simulink model "mech_car_kinematics"  (Simulink 7.1)
settings: Solver=ode45  StartTime=0.0  StopTime=10  RelTol=1e-3
PreLoadFcn:
  | % Initialize structures
  | chassis = struct() ;
  | wheelhub = struct() ;
  | suspension = struct() ;
  | wheel = struct() ;
  | 
  | % Defualt chassis/double wishbone mounting points
  | chassis.mass = 600 ;
  | chassis.upperfront = [0 0 0] ;
  | chassis.upperback = [-0.4 0 0] ;
  | chassis.lowerfront = [0 0 -0.5] ;
  | chassis.lowerback = [-0.4 0 -0.45] ;
  | chassis.steering = [0.12 0 -0.3] ;
  | chassis.suspension = [0 0 0.3] ;
  | 
  | % Default wheel hub/double wishbone mounting points
  | wheelhub.upper = [-0.2 0.55 0] ;
  | wheelhub.lower = [-0.2 0.55 -0.5] ;
  | wheelhub.steering = [0.05 0.5 -0.3] ;
  | wheelhub.suspension = [-0.2 0.55 -0.5] ;
  | 
  | % Default suspension parameters
  | suspension.ks = 16000 ;
  | suspension.bs = 1100 ;
  | suspension.Ls = 1.2 ;
  | 
  | % Defualt wheel parameters
  | wheel.radius = 0.3;
  | wheel.mass = 45 ;
  | wheel.inertia = [0.52 0 0;0 1 0;0 0 0.52]*2.5;
InitFcn:
  | set_param([gcs '/WORLD/Machine Environment'], 'AnalysisType', 'Kinematics');
StopFcn:
  | % Script to plot the bump steer properties of a suspension system
  | 
  | appDataName = 'mech_car_Kin_Steering_data';
  | figInfo.pos = [20   288   409   413];
  | figInfo.title = 'Steering angle versus CG height';
  | figInfo.xlabel = 'CG Height (m)';
  | figInfo.ylabel = 'Steering Angle (deg)';
  | mech_car_handling_fig_mgr('init',appDataName,figInfo);
  | modelFigure = getappdata(0,appDataName);
  | plot(-WHEEL.signals.values(:,1),STEER.signals.values,'Parent',modelFigure.axesH);
  | 
  | appDataName = 'mech_car_Kin_CamberAng_data';
  | figInfo.pos = [436   288   451   413];
  | figInfo.title = 'Camber angle versus CG height';
  | figInfo.xlabel = 'CG Height (m)';
  | figInfo.ylabel = 'Camber Angle (deg)';
  | mech_car_handling_fig_mgr('init',appDataName,figInfo);
  | modelFigure = getappdata(0,appDataName);
  | plot(-WHEEL.signals.values(:,1),CAMBER.signals.values,'Parent',modelFigure.axesH);
  | 
  | appDataName = 'mech_car_Kin_CasterAng_data';
  | figInfo.pos = [20   -154   411   369];
  | figInfo.title = 'Caster angle versus CG height';
  | figInfo.xlabel = 'CG Height (m)';
  | figInfo.ylabel = 'Caster Angle (deg)';
  | mech_car_handling_fig_mgr('init',appDataName,figInfo);
  | modelFigure = getappdata(0,appDataName);
  | plot(-WHEEL.signals.values(:,1),CASTER.signals.values,'Parent',modelFigure.axesH);
libraries: mblibv1 x27, mech_car_library x8, simulink x4
Description:
  | Car Suspension Kinematics
  | 
  | When designing a suspension system, it is important to know the effect of travel on the wheel alignment. This is measured by Camber, Steering, and Caster angles.
  | 
  | This quarter car model uses the SimMechanics Kinematics mode to measure these angles for a range of CG heights.
  | 
  | The Car parameters are defined in the PreLoad function of the model.
CloseFcn:
  | mech_car_handling_fig_mgr('destroy','mech_car_Kin_Steering_data');
  | mech_car_handling_fig_mgr('destroy','mech_car_Kin_CamberAng_data');
  | mech_car_handling_fig_mgr('destroy','mech_car_Kin_CasterAng_data');
settings Model: Creator=arnav  LastModifiedBy=batserve  BufferReuse=off
settings OptimizationCC: InlineParams=on  BufferReuse=off
settings DebuggingCC: SaveWithParameterizedLinksMsg=none  SignalResolutionControl=TryResolveAllWithWarning  SolverPrmCheckMsg=none  MultiTaskDSMMsg=warning  MultiTaskCondExecSysMsg=none  StrictBusMsg=None
settings HardwareCC: TargetBitPerLong=64  TargetEndianess=LittleEndian  TargetWordSize=64  TargetHWDeviceType=MATLAB Host  ProdEqTarget=off
settings RTWCC: SystemTargetFile=rsim.tlc  TemplateMakefile=rsim_default_tmf  Description=Rapid Simulation Target  ProcessScript=rsim_make_rtw_hook  IncludeERTFirstTime=on
settings RSimTargetCC: TargetFcnLib=ansi_tfl_tmw.mat  TargetFunctionLibrary=ANSI_C  IsPILTarget=off  EnableShiftOperators=on  PortableWordSizes=off
settings SimMechanicsCC: WarnOnRedundantConstraints=off  VisOnUpdateDiagram=on

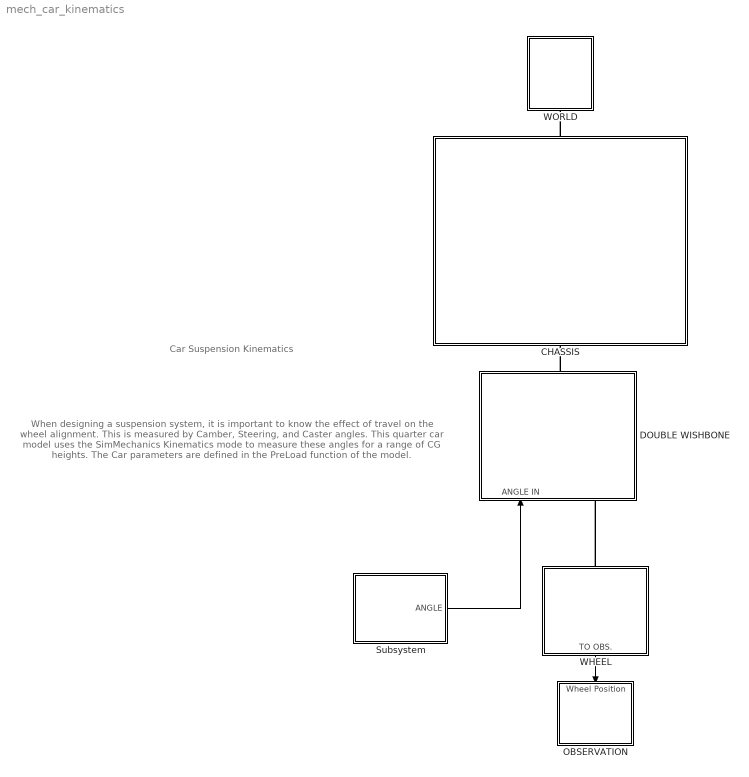
== system mech_car_kinematics ==
  note: When designing a suspension system, it is important
      | to know the effect of travel on the wheel alignment.
      | This is measured by Camber, Steering, and Caster angles.
      |
      | This quarter car model uses the SimMechanics Kinematics mode
      | to measure these angles for a range of CG heights.
      |
      | The Car parameters are defined in the PreLoad function of the model.
  note: Car Suspension Kinematics
  CHASSIS : Subsystem  Orientation=down  mask{chassis_mass=chassis.mass}
      mask prompts: chassis_mass "Quarter Car Chassis Mass"
      mask Display: image(imread('chassis.jpg'))
  DOUBLE WISHBONE : Subsystem  Orientation=up  mask{Chas_Up_Front=chassis.upperfront, Chas_Up_Back=chassis.upperback, Chas_Low_Front=chassis.lowerfront, Chas_Low_Back=chassis.lowerback, Chas_Steer=chassis.steering, Chas_Susp=chassis.suspension, Hub_Up=wheelhub.upper, Hub_Low=wheelhub.lower, Hub_Steer=wheelhub.steering, Hub_Susp=wheelhub.suspension, suspension_ks=suspension.ks, suspension_Ls=suspension.Ls, suspension_bs=suspension.bs}
      mask prompts: Chas_Up_Front "Chassis Upper Front Mounting"; Chas_Up_Back "Chassis Upper Back"; Chas_Low_Front "Chassis Lower Front"; Chas_Low_Back "Chassis Lower Back"; Chas_Steer "Chassis Steering Arm"; Chas_Susp "Chassis Suspension"; Hub_Up "Hub Upper"; Hub_Low "Hub Lower"; Hub_Steer "Hub Steering Arm"; Hub_Susp "Hub Suspension"; suspension_ks "Suspension Spring Stiffness"; suspension_Ls "Suspension Spring Natural Length"; suspension_bs "Suspension Damping Constant"
      mask Display: image(imread('double_wishbone.jpg'))
  OBSERVATION : Subsystem  Orientation=down
      mask Display: image(imread('view.jpg'))
  Subsystem : Subsystem
      mask Display: image(imread('spanner.jpg'))
  WHEEL : Subsystem  Orientation=down  mask{wheel_mass=wheel.mass, wheel_radius=wheel.radius, wheel_inertia=wheel.inertia}
      mask prompts: wheel_mass "Wheel Mass"; wheel_radius "Wheel Radius"; wheel_inertia "Wheel Inertia"
      mask Display: image(imread('wheel.jpg'))
  WORLD : Subsystem  Orientation=down
      mask Display: image(imread('sky.jpg'))
  wires:
  Subsystem/1(ANGLE) -> DOUBLE WISHBONE/1(ANGLE IN)
  WHEEL/1(TO OBS.) -> OBSERVATION/1(Wheel Position)
  connections:
  CHASSIS/LConn1 -- WORLD/RConn1
  WHEEL/LConn1 -- DOUBLE WISHBONE/LConn1
  DOUBLE WISHBONE/RConn1 -- CHASSIS/RConn1

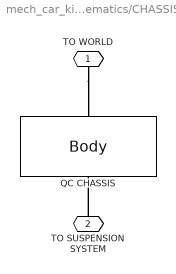
== system mech_car_kinematics/CHASSIS ==
  QC CHASSIS : mblibv1/Bodies/Body  Orientation=down  DialogController=MECH.DynMechDlgSource  PhysicalDomain=mechanical  SubClassName=Unknown  LeftPortType=workingframe  RightPortType=workingframe  LConnTagsString=CS1  RConnTagsString=CS2  DialogClass=MechanicalBodyBlock  Mass=chassis_mass  MassUnits=kg  InertiaUnits=kg*m^2  Inertia=diag([1 1 0.008])*10  Shape=Cylinder  ShapeDims=[1 1]  ShapeUnits=m  ShapeUse=false  Density=1  DensityUnits=kg/m^3  DensityUse=false  GraphicsMode=1  BodyColor=[0.5 0.5 0.5]  GraphicsObj=[]  AttachedToCS=1  CG=Left$CG$[0 0 -0.5]$CS1$CS1$m$[0 0 0]$EULER X-Y-Z$deg$WORLD$false  WorkingFrames=Left$CS1$[0 0 0]$ADJOINING$ADJOINING$m$[0 0 0]$EULER X-Y-Z$deg$WORLD$true#Right$CS2$[0 0 -1]$CS1$CS1$m$[0 0 0]$EULER X-Y-Z$deg$WORLD$true  CGPos=[0 0 -0.5]  CGRot=[0 0 0]  CS0Pos=[]  CS0Rot=[]  CS1Pos=[0 0 0]  CS1Rot=[0 0 0]  CS2Pos=[0 0 -1]  CS2Rot=[0 0 0]  CS3Pos=[]  CS3Rot=[]  CS4Pos=[]  CS4Rot=[]  CS5Pos=[]  CS5Rot=[]  CS6Pos=[]  CS6Rot=[]  CS7Pos=[]  CS7Rot=[]  CS8Pos=[]  CS8Rot=[]  CS9Pos=[]  CS9Rot=[]  CS10Pos=[]  CS10Rot=[]  CS11Pos=[]  CS11Rot=[]  CS12Pos=[]  CS12Rot=[]  CS13Pos=[]  CS13Rot=[]  CS14Pos=[]  CS14Rot=[]  CS15Pos=[]  CS15Rot=[]  CS16Pos=[]  CS16Rot=[]  CS17Pos=[]  CS17Rot=[]  CS18Pos=[]  CS18Rot=[]  CS19Pos=[]  CS19Rot=[]  CS20Pos=[]  CS20Rot=[]
  TO WORLD : PMIOPort  Orientation=down  Port=1  Side=Left
  TO SUSPENSION SYSTEM : PMIOPort  Orientation=up  Port=2  Side=Right
  connections:
  TO WORLD/RConn1 -- QC CHASSIS/LConn1
  TO SUSPENSION SYSTEM/RConn1 -- QC CHASSIS/RConn1

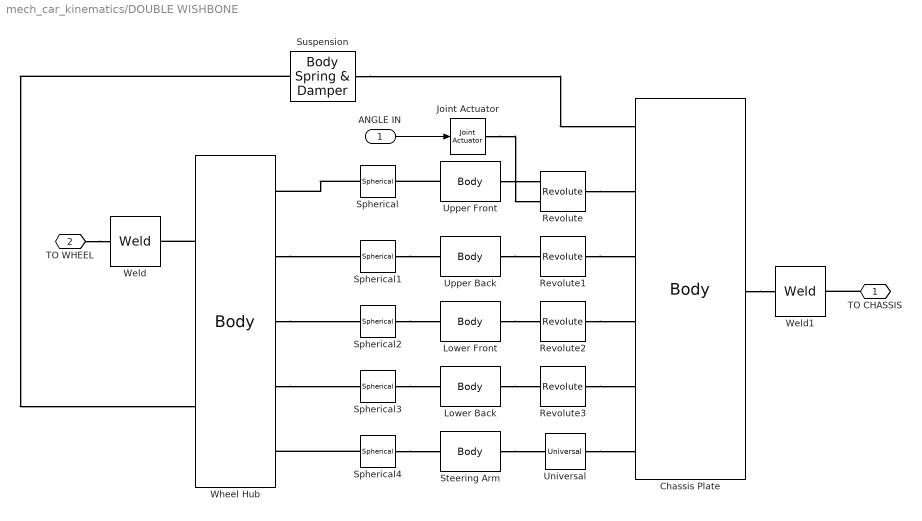
== system mech_car_kinematics/DOUBLE WISHBONE ==
  ANGLE IN : Inport  OutDataType=sfix(16)  OutScaling=2^0
  Chassis Plate : mblibv1/Bodies/Body  DialogController=MECH.DynMechDlgSource  PhysicalDomain=mechanical  SubClassName=Unknown  LeftPortType=workingframe  RightPortType=workingframe  LConnTagsString=CS1|CS3|CS2|CS5|CS6|CS7  RConnTagsString=CS4  DialogClass=MechanicalBodyBlock  Mass=0.1  MassUnits=kg  InertiaUnits=kg*m^2  Inertia=[0.5005 0 0;0 1 0;0 0 0.5005]/100  Shape=Cylinder  ShapeDims=[1 1]  ShapeUnits=m  ShapeUse=false  Density=1  DensityUnits=kg/m^3  DensityUse=false  GraphicsMode=1  BodyColor=[0.5 0.5 0.5]  GraphicsObj=[]  AttachedToCS=1  CG=Right$CG$[0 0 0]$CS4$CS4$m$[0 0 0]$EULER X-Y-Z$deg$WORLD$false  WorkingFrames=Right$CS4$[0 0 0]$ADJOINING$ADJOINING$m$[0 0 0]$EULER X-Y-Z$deg$WORLD$true#Left$CS1$Chas_Susp$CS4$CS4$m$[0 0 0]$EULER X-Y-Z$deg$WORLD$true#Left$CS3$Chas_Up_Front$CS4$CS4$m$[0 0 0]$EULER X-Y-Z$deg$WORLD$true#Left$CS2$Chas_Up_Back$CS4$CS4$m$[0 0 0]$EULER X-Y-Z$deg$WORLD$true#Left$CS5$Chas_Low_Front$CS4$CS4$m$[0 0 0]$EULER X-Y-Z$deg$WORLD$true#Left$CS6$Chas_Low_Back$CS4$CS4$m$[0 0 0]$EULER X-Y-Z$deg$WORLD$true#Left$CS7$Chas_Steer$CS4$CS4$m$[0 0 0]$EULER X-Y-Z$deg$WORLD$true  CGPos=[0 0 0]  CGRot=[0 0 0]  CS0Pos=[]  CS0Rot=[]  CS1Pos=Chas_Susp  CS1Rot=[0 0 0]  CS2Pos=Chas_Up_Back  CS2Rot=[0 0 0]  CS3Pos=Chas_Up_Front  CS3Rot=[0 0 0]  CS4Pos=[0 0 0]  CS4Rot=[0 0 0]  CS5Pos=Chas_Low_Front  CS5Rot=[0 0 0]  CS6Pos=Chas_Low_Back  CS6Rot=[0 0 0]  CS7Pos=Chas_Steer  CS7Rot=[0 0 0]  CS8Pos=[]  CS8Rot=[]  CS9Pos=[]  CS9Rot=[]  CS10Pos=[]  CS10Rot=[]  CS11Pos=[]  CS11Rot=[]  CS12Pos=[]  CS12Rot=[]  CS13Pos=[]  CS13Rot=[]  CS14Pos=[]  CS14Rot=[]  CS15Pos=[]  CS15Rot=[]  CS16Pos=[]  CS16Rot=[]  CS17Pos=[]  CS17Rot=[]  CS18Pos=[]  CS18Rot=[]  CS19Pos=[]  CS19Rot=[]  CS20Pos=[]  CS20Rot=[]
  Joint Actuator : mblibv1/Sensors &  Actuators/Joint Actuator  DialogController=MECH.DynMechDlgSource  SystemSampleTime=-1  PhysicalDomain=Mechanical  PortType=blob  ActuationStyle=Motion  AngleUnits=rad  ArcVelocityUnits=rad/s  ArcAccelerationUnits=rad/s^2  CoordPositionUnits=m  VelocityUnits=m/s  AccelerationUnits=m/s^2  ForceUnits=N  TorqueUnits=N-m  ActiveIO=on  Width=3  DialogClass=MechanicalActuatorBlock  Primitive=R1  ReferenceFrame=Absolute (INERTIAL)
  Lower Back : mblibv1/Bodies/Body  DialogController=MECH.DynMechDlgSource  PhysicalDomain=mechanical  SubClassName=Unknown  LeftPortType=workingframe  RightPortType=workingframe  LConnTagsString=CS1  RConnTagsString=CS2  DialogClass=MechanicalBodyBlock  Mass=7  MassUnits=kg  InertiaUnits=kg*m^2  Inertia=diag([0.008 1 1])/7.8  Shape=Cylinder  ShapeDims=[1 1]  ShapeUnits=m  ShapeUse=false  Density=1  DensityUnits=kg/m^3  DensityUse=false  GraphicsMode=1  BodyColor=[0.5 0.5 0.5]  GraphicsObj=[]  AttachedToCS=1  CG=Left$CG$0.5*(Hub_Low - Chas_Low_Back)$CS2$CS2$m$[0 0 -110]$EULER X-Y-Z$deg$WORLD$false  WorkingFrames=Left$CS1$Hub_Low - Chas_Low_Back$CS2$CS2$m$[0 0 0]$EULER X-Y-Z$deg$WORLD$true#Right$CS2$[0 0 0]$ADJOINING$ADJOINING$m$[0 0 0]$EULER X-Y-Z$deg$WORLD$true  CGPos=0.5*(Hub_Low - Chas_Low_Back)  CGRot=[0 0 -110]  CS0Pos=[]  CS0Rot=[]  CS1Pos=Hub_Low - Chas_Low_Back  CS1Rot=[0 0 0]  CS2Pos=[0 0 0]  CS2Rot=[0 0 0]  CS3Pos=[]  CS3Rot=[]  CS4Pos=[]  CS4Rot=[]  CS5Pos=[]  CS5Rot=[]  CS6Pos=[]  CS6Rot=[]  CS7Pos=[]  CS7Rot=[]  CS8Pos=[]  CS8Rot=[]  CS9Pos=[]  CS9Rot=[]  CS10Pos=[]  CS10Rot=[]  CS11Pos=[]  CS11Rot=[]  CS12Pos=[]  CS12Rot=[]  CS13Pos=[]  CS13Rot=[]  CS14Pos=[]  CS14Rot=[]  CS15Pos=[]  CS15Rot=[]  CS16Pos=[]  CS16Rot=[]  CS17Pos=[]  CS17Rot=[]  CS18Pos=[]  CS18Rot=[]  CS19Pos=[]  CS19Rot=[]  CS20Pos=[]  CS20Rot=[]
  Lower Front : mblibv1/Bodies/Body  DialogController=MECH.DynMechDlgSource  PhysicalDomain=mechanical  SubClassName=Unknown  LeftPortType=workingframe  RightPortType=workingframe  LConnTagsString=CS1  RConnTagsString=CS2  DialogClass=MechanicalBodyBlock  Mass=7  MassUnits=kg  InertiaUnits=kg*m^2  Inertia=diag([0.008 1 1])/7.8  Shape=Cylinder  ShapeDims=[1 1]  ShapeUnits=m  ShapeUse=false  Density=1  DensityUnits=kg/m^3  DensityUse=false  GraphicsMode=1  BodyColor=[0.5 0.5 0.5]  GraphicsObj=[]  AttachedToCS=1  CG=Left$CG$0.5*(Hub_Low - Chas_Low_Front)$CS2$CS2$m$[0 0 -70]$EULER X-Y-Z$deg$WORLD$false  WorkingFrames=Left$CS1$Hub_Low - Chas_Low_Front$CS2$CS2$m$[0 0 0]$EULER X-Y-Z$deg$WORLD$true#Right$CS2$[0 0 0]$ADJOINING$ADJOINING$m$[0 0 0]$EULER X-Y-Z$deg$WORLD$true  CGPos=0.5*(Hub_Low - Chas_Low_Front)  CGRot=[0 0 -70]  CS0Pos=[]  CS0Rot=[]  CS1Pos=Hub_Low - Chas_Low_Front  CS1Rot=[0 0 0]  CS2Pos=[0 0 0]  CS2Rot=[0 0 0]  CS3Pos=[]  CS3Rot=[]  CS4Pos=[]  CS4Rot=[]  CS5Pos=[]  CS5Rot=[]  CS6Pos=[]  CS6Rot=[]  CS7Pos=[]  CS7Rot=[]  CS8Pos=[]  CS8Rot=[]  CS9Pos=[]  CS9Rot=[]  CS10Pos=[]  CS10Rot=[]  CS11Pos=[]  CS11Rot=[]  CS12Pos=[]  CS12Rot=[]  CS13Pos=[]  CS13Rot=[]  CS14Pos=[]  CS14Rot=[]  CS15Pos=[]  CS15Rot=[]  CS16Pos=[]  CS16Rot=[]  CS17Pos=[]  CS17Rot=[]  CS18Pos=[]  CS18Rot=[]  CS19Pos=[]  CS19Rot=[]  CS20Pos=[]  CS20Rot=[]
  Revolute : mblibv1/Joints/Revolute  DialogController=MECH.DynMechDlgSource  PhysicalDomain=mechanical  SubClassName=Unknown  LeftPortType=blob  RightPortType=blob  LConnTagsString=__newl0|SA1  RConnTagsString=__newr0  NumSAPorts=1  CutJoint=off  MarkAsCut=off  Primitives=revolute  PrimitiveProps=R1$WORLD$Chas_Up_Front - Chas_Up_Back$revolute  DialogClass=JointBlock  R1Axis=Chas_Up_Front - Chas_Up_Back
  Revolute1 : mblibv1/Joints/Revolute  DialogController=MECH.DynMechDlgSource  PhysicalDomain=mechanical  SubClassName=Unknown  LeftPortType=blob  RightPortType=blob  LConnTagsString=__newl0  RConnTagsString=__newr0  NumSAPorts=0  CutJoint=on  MarkAsCut=off  Primitives=revolute  PrimitiveProps=R1$WORLD$Chas_Up_Front - Chas_Up_Back$revolute  DialogClass=JointBlock  R1Axis=Chas_Up_Front - Chas_Up_Back
  Revolute2 : mblibv1/Joints/Revolute  DialogController=MECH.DynMechDlgSource  PhysicalDomain=mechanical  SubClassName=Unknown  LeftPortType=blob  RightPortType=blob  LConnTagsString=__newl0  RConnTagsString=__newr0  NumSAPorts=0  CutJoint=off  MarkAsCut=off  Primitives=revolute  PrimitiveProps=R1$WORLD$Chas_Low_Front-Chas_Low_Back$revolute  DialogClass=JointBlock  R1Axis=Chas_Low_Front-Chas_Low_Back
  Revolute3 : mblibv1/Joints/Revolute  DialogController=MECH.DynMechDlgSource  PhysicalDomain=mechanical  SubClassName=Unknown  LeftPortType=blob  RightPortType=blob  LConnTagsString=__newl0  RConnTagsString=__newr0  NumSAPorts=0  CutJoint=off  MarkAsCut=off  Primitives=revolute  PrimitiveProps=R1$WORLD$Chas_Low_Front - Chas_Low_Back$revolute  DialogClass=JointBlock  R1Axis=Chas_Low_Front - Chas_Low_Back
  Spherical : mblibv1/Joints/Spherical  DialogController=MECH.DynMechDlgSource  PhysicalDomain=mechanical  SubClassName=Unknown  LeftPortType=blob  RightPortType=blob  LConnTagsString=__newl0  RConnTagsString=__newr0  NumSAPorts=0  CutJoint=off  MarkAsCut=off  Primitives=spherical  PrimitiveProps=S$INERTIAL$[0 0 0]$spherical  DialogClass=JointBlock  SAxis=[0 0 0]
  Spherical1 : mblibv1/Joints/Spherical  DialogController=MECH.DynMechDlgSource  PhysicalDomain=mechanical  SubClassName=Unknown  LeftPortType=blob  RightPortType=blob  LConnTagsString=__newl0  RConnTagsString=__newr0  NumSAPorts=0  CutJoint=off  MarkAsCut=off  Primitives=spherical  PrimitiveProps=S$WORLD$[0 0 0]$spherical  DialogClass=JointBlock  SAxis=[0 0 0]
  Spherical2 : mblibv1/Joints/Spherical  DialogController=MECH.DynMechDlgSource  PhysicalDomain=mechanical  SubClassName=Unknown  LeftPortType=blob  RightPortType=blob  LConnTagsString=__newl0  RConnTagsString=__newr0  NumSAPorts=0  CutJoint=off  MarkAsCut=off  Primitives=spherical  PrimitiveProps=S$WORLD$[0 0 0]$spherical  DialogClass=JointBlock  SAxis=[0 0 0]
  Spherical3 : mblibv1/Joints/Spherical  DialogController=MECH.DynMechDlgSource  PhysicalDomain=mechanical  SubClassName=Unknown  LeftPortType=blob  RightPortType=blob  LConnTagsString=__newl0  RConnTagsString=__newr0  NumSAPorts=0  CutJoint=on  MarkAsCut=off  Primitives=spherical  PrimitiveProps=S$WORLD$[0 0 0]$spherical  DialogClass=JointBlock  SAxis=[0 0 0]
  Spherical4 : mblibv1/Joints/Spherical  DialogController=MECH.DynMechDlgSource  PhysicalDomain=mechanical  SubClassName=Unknown  LeftPortType=blob  RightPortType=blob  LConnTagsString=__newl0  RConnTagsString=__newr0  NumSAPorts=0  CutJoint=off  MarkAsCut=off  Primitives=spherical  PrimitiveProps=S$INERTIAL$[0 0 0]$spherical  DialogClass=JointBlock  SAxis=[0 0 0]
  Steering Arm : mblibv1/Bodies/Body  DialogController=MECH.DynMechDlgSource  PhysicalDomain=mechanical  SubClassName=Unknown  LeftPortType=workingframe  RightPortType=workingframe  LConnTagsString=CS1  RConnTagsString=CS2  DialogClass=MechanicalBodyBlock  Mass=7  MassUnits=kg  InertiaUnits=kg*m^2  Inertia=diag([0.008 1 1])/10  Shape=Cylinder  ShapeDims=[1 1]  ShapeUnits=m  ShapeUse=false  Density=1  DensityUnits=kg/m^3  DensityUse=false  GraphicsMode=1  BodyColor=[0.5 0.5 0.5]  GraphicsObj=[]  AttachedToCS=1  CG=Left$CG$0.5*(Hub_Steer - Chas_Steer)$CS2$CS2$m$[0 0 -82]$EULER X-Y-Z$deg$WORLD$false  WorkingFrames=Left$CS1$Hub_Steer - Chas_Steer$CS2$CS2$m$[0 0 0]$EULER X-Y-Z$deg$WORLD$true#Right$CS2$[0 0 0]$ADJOINING$ADJOINING$m$[0 0 0]$EULER X-Y-Z$deg$WORLD$true  CGPos=0.5*(Hub_Steer - Chas_Steer)  CGRot=[0 0 -82]  CS0Pos=[]  CS0Rot=[]  CS1Pos=Hub_Steer - Chas_Steer  CS1Rot=[0 0 0]  CS2Pos=[0 0 0]  CS2Rot=[0 0 0]  CS3Pos=[]  CS3Rot=[]  CS4Pos=[]  CS4Rot=[]  CS5Pos=[]  CS5Rot=[]  CS6Pos=[]  CS6Rot=[]  CS7Pos=[]  CS7Rot=[]  CS8Pos=[]  CS8Rot=[]  CS9Pos=[]  CS9Rot=[]  CS10Pos=[]  CS10Rot=[]  CS11Pos=[]  CS11Rot=[]  CS12Pos=[]  CS12Rot=[]  CS13Pos=[]  CS13Rot=[]  CS14Pos=[]  CS14Rot=[]  CS15Pos=[]  CS15Rot=[]  CS16Pos=[]  CS16Rot=[]  CS17Pos=[]  CS17Rot=[]  CS18Pos=[]  CS18Rot=[]  CS19Pos=[]  CS19Rot=[]  CS20Pos=[]  CS20Rot=[]
  Suspension : mblibv1/Force  Elements/Body Spring & Damper  DialogController=MECH.DynMechDlgSource  SystemSampleTime=-1  DialogClass=BodySpringDamper  Spring_k=suspension_ks  Damper_b=suspension_bs  Offset_x0=suspension_Ls  PositionUnits=m  VelocityUnits=m/s  ForceUnits=N
  Universal : mblibv1/Joints/Universal  DialogController=MECH.DynMechDlgSource  PhysicalDomain=mechanical  SubClassName=Unknown  LeftPortType=blob  RightPortType=blob  LConnTagsString=__newl0  RConnTagsString=__newr0  NumSAPorts=0  CutJoint=off  MarkAsCut=off  Primitives=revolute_revolute  PrimitiveProps=R1$WORLD$[1 0 0]$revolute#R2$WORLD$[0 0 1]$revolute  DialogClass=JointBlock  R1Axis=[1 0 0]  R2Axis=[0 0 1]
  Upper Back : mblibv1/Bodies/Body  DialogController=MECH.DynMechDlgSource  PhysicalDomain=mechanical  SubClassName=Unknown  LeftPortType=workingframe  RightPortType=workingframe  LConnTagsString=CS1  RConnTagsString=CS2  DialogClass=MechanicalBodyBlock  Mass=7  MassUnits=kg  InertiaUnits=kg*m^2  Inertia=diag([0.008 1 1])/7.8  Shape=Cylinder  ShapeDims=[1 1]  ShapeUnits=m  ShapeUse=false  Density=1  DensityUnits=kg/m^3  DensityUse=false  GraphicsMode=1  BodyColor=[0.5 0.5 0.5]  GraphicsObj=[]  AttachedToCS=1  CG=Left$CG$0.5*(Hub_Up - Chas_Up_Back)$CS2$CS2$m$[0 0 -110]$EULER X-Y-Z$deg$WORLD$false  WorkingFrames=Left$CS1$(Hub_Up - Chas_Up_Back)$CS2$CS2$m$[0 0 0]$EULER X-Y-Z$deg$WORLD$true#Right$CS2$[0 0 0]$ADJOINING$ADJOINING$m$[0 0 0]$EULER X-Y-Z$deg$WORLD$true  CGPos=0.5*(Hub_Up - Chas_Up_Back)  CGRot=[0 0 -110]  CS0Pos=[]  CS0Rot=[]  CS1Pos=(Hub_Up - Chas_Up_Back)  CS1Rot=[0 0 0]  CS2Pos=[0 0 0]  CS2Rot=[0 0 0]  CS3Pos=[]  CS3Rot=[]  CS4Pos=[]  CS4Rot=[]  CS5Pos=[]  CS5Rot=[]  CS6Pos=[]  CS6Rot=[]  CS7Pos=[]  CS7Rot=[]  CS8Pos=[]  CS8Rot=[]  CS9Pos=[]  CS9Rot=[]  CS10Pos=[]  CS10Rot=[]  CS11Pos=[]  CS11Rot=[]  CS12Pos=[]  CS12Rot=[]  CS13Pos=[]  CS13Rot=[]  CS14Pos=[]  CS14Rot=[]  CS15Pos=[]  CS15Rot=[]  CS16Pos=[]  CS16Rot=[]  CS17Pos=[]  CS17Rot=[]  CS18Pos=[]  CS18Rot=[]  CS19Pos=[]  CS19Rot=[]  CS20Pos=[]  CS20Rot=[]
  Upper Front : mblibv1/Bodies/Body  DialogController=MECH.DynMechDlgSource  PhysicalDomain=mechanical  SubClassName=Unknown  LeftPortType=workingframe  RightPortType=workingframe  LConnTagsString=CS1  RConnTagsString=CS2  DialogClass=MechanicalBodyBlock  Mass=7  MassUnits=kg  InertiaUnits=kg*m^2  Inertia=diag([0.008 1 1])/7.8  Shape=Cylinder  ShapeDims=[1 1]  ShapeUnits=m  ShapeUse=false  Density=1  DensityUnits=kg/m^3  DensityUse=false  GraphicsMode=1  BodyColor=[0.5 0.5 0.5]  GraphicsObj=[]  AttachedToCS=1  CG=Left$CG$[-0.1 0.25 0]$CS2$CS2$m$[0 0 -70]$EULER X-Y-Z$deg$WORLD$false  WorkingFrames=Left$CS1$Hub_Up - Chas_Up_Front$CS2$CS2$m$[0 0 0]$EULER X-Y-Z$deg$WORLD$true#Right$CS2$[0 0 0]$ADJOINING$ADJOINING$m$[0 0 0]$EULER X-Y-Z$deg$WORLD$true  CGPos=[-0.1 0.25 0]  CGRot=[0 0 -70]  CS0Pos=[]  CS0Rot=[]  CS1Pos=Hub_Up - Chas_Up_Front  CS1Rot=[0 0 0]  CS2Pos=[0 0 0]  CS2Rot=[0 0 0]  CS3Pos=[]  CS3Rot=[]  CS4Pos=[]  CS4Rot=[]  CS5Pos=[]  CS5Rot=[]  CS6Pos=[]  CS6Rot=[]  CS7Pos=[]  CS7Rot=[]  CS8Pos=[]  CS8Rot=[]  CS9Pos=[]  CS9Rot=[]  CS10Pos=[]  CS10Rot=[]  CS11Pos=[]  CS11Rot=[]  CS12Pos=[]  CS12Rot=[]  CS13Pos=[]  CS13Rot=[]  CS14Pos=[]  CS14Rot=[]  CS15Pos=[]  CS15Rot=[]  CS16Pos=[]  CS16Rot=[]  CS17Pos=[]  CS17Rot=[]  CS18Pos=[]  CS18Rot=[]  CS19Pos=[]  CS19Rot=[]  CS20Pos=[]  CS20Rot=[]
  Weld : mblibv1/Joints/Weld  DialogController=MECH.DynMechDlgSource  PhysicalDomain=mechanical  SubClassName=Unknown  LeftPortType=blob  RightPortType=blob  LConnTagsString=__newl0  RConnTagsString=__newr0  NumSAPorts=0  CutJoint=off  MarkAsCut=off  Primitives=weld  PrimitiveProps=W$INERTIAL$[0 0 0]$weld  DialogClass=JointBlock  WAxis=[0 0 0]
  Weld1 : mblibv1/Joints/Weld  DialogController=MECH.DynMechDlgSource  PhysicalDomain=mechanical  SubClassName=Unknown  LeftPortType=blob  RightPortType=blob  LConnTagsString=__newl0  RConnTagsString=__newr0  NumSAPorts=0  CutJoint=off  MarkAsCut=off  Primitives=weld  PrimitiveProps=W$INERTIAL$[0 0 0]$weld  DialogClass=JointBlock  WAxis=[0 0 0]
  Wheel Hub : mblibv1/Bodies/Body  DialogController=MECH.DynMechDlgSource  PhysicalDomain=mechanical  SubClassName=Unknown  LeftPortType=workingframe  RightPortType=workingframe  LConnTagsString=CS1|CS2  RConnTagsString=CS3|CS6|CS4|CS5|CS7  DialogClass=MechanicalBodyBlock  Mass=5  MassUnits=kg  InertiaUnits=kg*m^2  Inertia=[0.55 0 0;0 1 0;0 0 0.55]/12  Shape=Cylinder  ShapeDims=[1 1]  ShapeUnits=m  ShapeUse=false  Density=1  DensityUnits=kg/m^3  DensityUse=false  GraphicsMode=1  BodyColor=[0.5 0.5 0.5]  GraphicsObj=[]  AttachedToCS=1  CG=Left$CG$[0 0.03 -0.2]$CS3$CS3$m$[0 0 0]$EULER X-Y-Z$deg$WORLD$false  WorkingFrames=Left$CS1$[0 0.1 -0.2]$CS3$CS3$m$[0 0 0]$EULER X-Y-Z$deg$WORLD$true#Right$CS3$Hub_Up - [0 0 1]$WORLD$WORLD$m$[0 0 0]$EULER X-Y-Z$deg$WORLD$true#Right$CS6$Hub_Up - [0 0 1]$WORLD$WORLD$m$[0 0 0]$EULER X-Y-Z$deg$WORLD$true#Left$CS2$Hub_Susp - [0 0 1]$WORLD$WORLD$m$[0 0 0]$EULER X-Y-Z$deg$WORLD$true#Right$CS4$Hub_Low - [0 0 1]$WORLD$WORLD$m$[0 0 0]$EULER X-Y-Z$deg$WORLD$true#Right$CS5$Hub_Low - [0 0 1]$WORLD$WORLD$m$[0 0 0]$EULER X-Y-Z$deg$WORLD$true#Right$CS7$Hub_Steer - [0 0 1]$WORLD$WORLD$m$[0 0 0]$EULER X-Y-Z$deg$WORLD$true  CGPos=[0 0.03 -0.2]  CGRot=[0 0 0]  CS0Pos=[]  CS0Rot=[]  CS1Pos=[0 0.1 -0.2]  CS1Rot=[0 0 0]  CS2Pos=Hub_Susp - [0 0 1]  CS2Rot=[0 0 0]  CS3Pos=Hub_Up - [0 0 1]  CS3Rot=[0 0 0]  CS4Pos=Hub_Low - [0 0 1]  CS4Rot=[0 0 0]  CS5Pos=Hub_Low - [0 0 1]  CS5Rot=[0 0 0]  CS6Pos=Hub_Up - [0 0 1]  CS6Rot=[0 0 0]  CS7Pos=Hub_Steer - [0 0 1]  CS7Rot=[0 0 0]  CS8Pos=[]  CS8Rot=[]  CS9Pos=[]  CS9Rot=[]  CS10Pos=[]  CS10Rot=[]  CS11Pos=[]  CS11Rot=[]  CS12Pos=[]  CS12Rot=[]  CS13Pos=[]  CS13Rot=[]  CS14Pos=[]  CS14Rot=[]  CS15Pos=[]  CS15Rot=[]  CS16Pos=[]  CS16Rot=[]  CS17Pos=[]  CS17Rot=[]  CS18Pos=[]  CS18Rot=[]  CS19Pos=[]  CS19Rot=[]  CS20Pos=[]  CS20Rot=[]
  TO CHASSIS : PMIOPort  Orientation=left  Port=1  Side=Right
  TO WHEEL : PMIOPort  Port=2  Side=Left
  wires:
  ANGLE IN/1 -> Joint Actuator/1
  connections:
  Suspension/RConn1 -- Chassis Plate/LConn1
  Revolute/RConn1 -- Chassis Plate/LConn2
  Chassis Plate/RConn1 -- Weld1/LConn1
  Spherical3/RConn1 -- Lower Back/LConn1
  Lower Back/RConn1 -- Revolute3/LConn1
  Spherical2/RConn1 -- Lower Front/LConn1
  Lower Front/RConn1 -- Revolute2/LConn1
  Upper Front/RConn1 -- Revolute/LConn1
  Upper Back/RConn1 -- Revolute1/LConn1
  Spherical/LConn1 -- Wheel Hub/RConn1
  Upper Front/LConn1 -- Spherical/RConn1
  Wheel Hub/RConn2 -- Spherical1/LConn1
  Spherical1/RConn1 -- Upper Back/LConn1
  Wheel Hub/RConn3 -- Spherical2/LConn1
  Wheel Hub/RConn4 -- Spherical3/LConn1
  Wheel Hub/LConn1 -- Weld/RConn1
  TO CHASSIS/RConn1 -- Weld1/RConn1
  TO WHEEL/RConn1 -- Weld/LConn1
  Universal/RConn1 -- Chassis Plate/LConn6
  Spherical4/LConn1 -- Wheel Hub/RConn5
  Spherical4/RConn1 -- Steering Arm/LConn1
  Steering Arm/RConn1 -- Universal/LConn1
  Joint Actuator/RConn1 -- Revolute/LConn2
  Revolute3/RConn1 -- Chassis Plate/LConn5
  Revolute2/RConn1 -- Chassis Plate/LConn4
  Revolute1/RConn1 -- Chassis Plate/LConn3
  Suspension/LConn1 -- Wheel Hub/LConn2

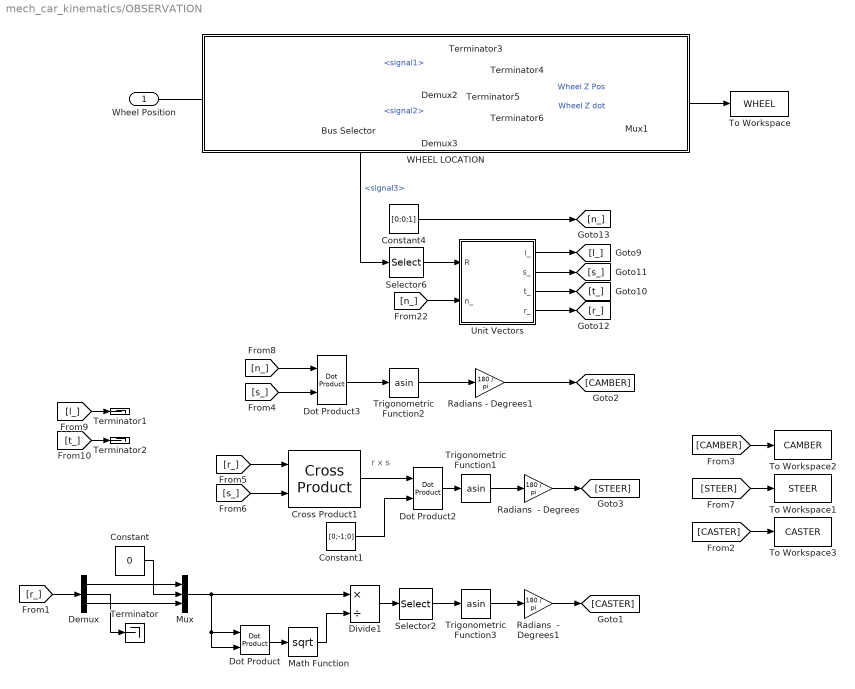
== system mech_car_kinematics/OBSERVATION ==
  note: r x s
  Wheel Position : Inport  OutDataType=sfix(16)  OutScaling=2^0
  Bus Selector : BusSelector  OutputSignals=signal1,signal2,signal3
  Constant : Constant  Value=0  OutDataType=sfix(16)  OutScaling=2^0
  Constant1 : Constant  Value=[0;-1;0]  OutDataType=sfix(16)  OutScaling=2^0
  Constant4 : Constant  Value=[0;0;1]  OutDataType=sfix(16)  OutScaling=2^0
  Cross Product1 : mech_car_library/Utilities/Cross Product  SystemSampleTime=-1
  Demux : Demux  Outputs=3
  Demux2 : Demux  Outputs=3
  Demux3 : Demux  Outputs=3
  Divide1 : Product  Inputs=*/  OutDataType=sfix(16)  OutScaling=2^-10
  Dot Product : simulink/Math Operations/Dot Product  InputSameDT=on  OutDataType=sfix(16)  OutScaling=2^-10  DoSatur=off
  Dot Product2 : simulink/Math Operations/Dot Product  InputSameDT=on  OutDataType=sfix(16)  OutScaling=2^-10  DoSatur=off
  Dot Product3 : simulink/Math Operations/Dot Product  InputSameDT=on  OutDataType=sfix(16)  OutScaling=2^-10  DoSatur=off
  Math Function : Math  Operator=sqrt  OutDataType=sfix(16)  OutScaling=2^0  SaturateOnIntegerOverflow=on
  Mux : Mux  Inputs=3
  Mux1 : Mux  Inputs=2
  Radians  - Degrees : Gain  Gain=180 / pi  ParameterDataType=sfix(16)  ParameterScaling=2^0  OutDataType=sfix(16)  OutScaling=2^0
  Radians  - Degrees1 : Gain  Gain=180 / pi  ParameterDataType=sfix(16)  ParameterScaling=2^0  OutDataType=sfix(16)  OutScaling=2^0
  Radians - Degrees1 : Gain  Gain=180 / pi  ParameterDataType=sfix(16)  ParameterScaling=2^0  OutDataType=sfix(16)  OutScaling=2^0
  Selector2 : Selector  InputPortWidth=3  IndexOptions=Index vector (dialog)  Indices=1  OutputSizes=1
  Selector6 : Selector  InputPortWidth=9  IndexOptions=Index vector (dialog)  Indices=1:9  OutputSizes=1
  Terminator{,1..6} (7 alike) : Terminator
  To Workspace : ToWorkspace  VariableName=WHEEL  SampleTime=-1  SaveFormat=Structure
  To Workspace1 : ToWorkspace  VariableName=STEER  SampleTime=-1  SaveFormat=Structure
  To Workspace2 : ToWorkspace  VariableName=CAMBER  SampleTime=-1  SaveFormat=Structure
  To Workspace3 : ToWorkspace  VariableName=CASTER  SampleTime=-1  SaveFormat=Structure
  Trigonometric Function1 : Trigonometry  Operator=asin
  Trigonometric Function2 : Trigonometry  Operator=asin
  Trigonometric Function3 : Trigonometry  Operator=asin
  Unit Vectors : Subsystem
  WHEEL LOCATION : Subsystem
      mask Display: disp('')
  wires:
  Bus Selector/1 -> Demux2/1  "<signal1>"
  Bus Selector/2 -> Demux3/1  "<signal2>"
  Demux2/2 -> Terminator4/1
  Demux2/3 -> Mux1/1  "Wheel Z Pos"
  Demux3/3 -> Mux1/2  "Wheel Z dot"
  Demux3/1 -> Terminator5/1
  Demux3/2 -> Terminator6/1
  Bus Selector/3 -> Selector6/1  "<signal3>"
  [n_] -> Unit Vectors/2(n_)
  Constant4/1 -> [n_]
  Unit Vectors/3(t_) -> [t_]
  Unit Vectors/4(r_) -> [r_]
  Unit Vectors/2(s_) -> [s_]
  Unit Vectors/1(l_) -> [l_]
  Selector6/1 -> Unit Vectors/1(R)
  [r_] -> Cross Product1/1
  [s_] -> Cross Product1/2
  Cross Product1/1 -> Dot Product2/1
  Constant1/1 -> Dot Product2/2
  Dot Product2/1 -> Trigonometric Function1/1
  Radians  - Degrees/1 -> [STEER]
  [l_] -> Terminator1/1
  [t_] -> Terminator2/1
  Wheel Position/1 -> Bus Selector/1
  [CAMBER] -> To Workspace2/1
  [STEER] -> To Workspace1/1
  Trigonometric Function1/1 -> Radians  - Degrees/1
  Demux2/1 -> Terminator3/1
  Mux1/1 -> To Workspace/1
  [n_] -> Dot Product3/1
  [s_] -> Dot Product3/2
  Dot Product3/1 -> Trigonometric Function2/1
  Trigonometric Function2/1 -> Radians - Degrees1/1
  Radians - Degrees1/1 -> [CAMBER]
  [r_] -> Demux/1
  Demux/1 -> Mux/1
  Demux/3 -> Mux/3
  Demux/2 -> Terminator/1
  Constant/1 -> Mux/2
  Mux/1 -> Dot Product/1, Dot Product/2, Divide1/1
  Dot Product/1 -> Math Function/1
  Math Function/1 -> Divide1/2
  Divide1/1 -> Selector2/1
  Selector2/1 -> Trigonometric Function3/1
  Trigonometric Function3/1 -> Radians  - Degrees1/1
  [CASTER] -> To Workspace3/1
  Radians  - Degrees1/1 -> [CASTER]

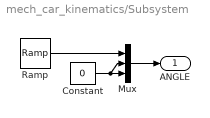
== system mech_car_kinematics/Subsystem ==
  Constant : Constant  Value=0  OutDataType=sfix(16)  OutScaling=2^0
  Mux : Mux  Inputs=3
  Ramp : simulink/Sources/Ramp  SystemSampleTime=-1  slope=0.1  start=0  X0=-0.5
  ANGLE : Outport  OutDataType=sfix(16)  OutScaling=2^0
  wires:
  Ramp/1 -> Mux/1
  Constant/1 -> Mux/2, Mux/3
  Mux/1 -> ANGLE/1

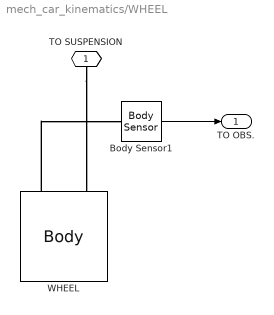
== system mech_car_kinematics/WHEEL ==
  Body Sensor1 : mblibv1/Sensors &  Actuators/Body Sensor  DialogController=MECH.DynMechDlgSource  SystemSampleTime=-1  PhysicalDomain=Mechanical  PortType=blob  Muxed=on  Pose=on  Angle=on  AngleUnits=deg  ArcVelocity=off  ArcVelocityUnits=deg/s  ArcAcceleration=off  ArcAccelerationUnits=deg/s^2  CoordPosition=on  CoordPositionUnits=m  Velocity=on  VelocityUnits=m/s  Acceleration=off  AccelerationUnits=m/s^2  Quaternion=on  QuaternionDT=off  QuaternionDDT=off  QuaternionUnits=off  OutputVector=[ 3 3 9 ]  ActiveIO=on  Width=15  DialogClass=MechanicalSensorBlock  ReferenceFrame=Absolute (World)
  WHEEL : mblibv1/Bodies/Body  Orientation=down  DialogController=MECH.DynMechDlgSource  PhysicalDomain=mechanical  SubClassName=Unknown  LeftPortType=workingframe  RightPortType=workingframe  LConnTagsString=CG|CS1  DialogClass=MechanicalBodyBlock  Mass=wheel_mass  MassUnits=kg  InertiaUnits=kg*m^2  Inertia=wheel_inertia  Shape=Cylinder  ShapeDims=[1 1]  ShapeUnits=m  ShapeUse=false  Density=1  DensityUnits=kg/m^3  DensityUse=false  GraphicsMode=1  BodyColor=[0.5 0.5 0.5]  GraphicsObj=[]  AttachedToCS=1  CG=Left$CG$[0 0 0]$CS1$CS1$m$[0 0 0]$EULER X-Y-Z$deg$WORLD$true  WorkingFrames=Left$CS1$[0 0 0]$ADJOINING$ADJOINING$m$[0 0 0]$EULER X-Y-Z$deg$WORLD$true#Right$CS2$[0 0 -wheel_radius]$CS1$CS1$m$[0 0 0]$EULER X-Y-Z$deg$WORLD$false#Right$CS3$[wheel_radius 0 0]$CS1$CS1$m$[0 0 0]$EULER X-Y-Z$deg$WORLD$false#Right$CS4$-[wheel_radius 0 0]$CS1$CS1$m$[0 0 0]$EULER X-Y-Z$deg$WORLD$false  CGPos=[0 0 0]  CGRot=[0 0 0]  CS0Pos=[]  CS0Rot=[]  CS1Pos=[0 0 0]  CS1Rot=[0 0 0]  CS2Pos=[0 0 -wheel_radius]  CS2Rot=[0 0 0]  CS3Pos=[wheel_radius 0 0]  CS3Rot=[0 0 0]  CS4Pos=-[wheel_radius 0 0]  CS4Rot=[0 0 0]  CS5Pos=[]  CS5Rot=[]  CS6Pos=[]  CS6Rot=[]  CS7Pos=[]  CS7Rot=[]  CS8Pos=[]  CS8Rot=[]  CS9Pos=[]  CS9Rot=[]  CS10Pos=[]  CS10Rot=[]  CS11Pos=[]  CS11Rot=[]  CS12Pos=[]  CS12Rot=[]  CS13Pos=[]  CS13Rot=[]  CS14Pos=[]  CS14Rot=[]  CS15Pos=[]  CS15Rot=[]  CS16Pos=[]  CS16Rot=[]  CS17Pos=[]  CS17Rot=[]  CS18Pos=[]  CS18Rot=[]  CS19Pos=[]  CS19Rot=[]  CS20Pos=[]  CS20Rot=[]
  TO SUSPENSION : PMIOPort  Orientation=down  Port=1  Side=Left
  TO OBS. : Outport  OutDataType=sfix(16)  OutScaling=2^0
  wires:
  Body Sensor1/1 -> TO OBS./1
  connections:
  TO SUSPENSION/RConn1 -- WHEEL/LConn2
  WHEEL/LConn1 -- Body Sensor1/LConn1

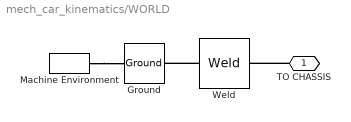
== system mech_car_kinematics/WORLD ==
  Ground : mblibv1/Bodies/Ground  DialogController=MECH.DynMechDlgSource  SystemSampleTime=-1  LeftPortType=env  RightPortType=workingframe  PhysicalDomain=Mechanical  DialogClass=GroundBlock  CoordPosition=[0 0 0]  CoordPositionUnits=m  StateVectorMgrId=-1  MachineId=[0 0]  ShowEnvPort=on
  Machine Environment : mblibv1/Bodies/Machine Environment  Tag=Factory ground  DialogController=MECH.DialogSource  SystemSampleTime=-1  PortType=env  PhysicalDomain=Mechanical  DialogTemplateClass=MECH.MachineEnvironment  SyncWhenCopied=off  Gravity=[0 0 -9.81]  GravityUnits=m/s^2  GravityAsSignal=off  Dimensionality=Auto-detect  AnalysisType=Kinematics  LinearAssemblyTolerance=1e-3  LinearAssemblyToleranceUnits=m  AngularAssemblyTolerance=1e-3  AngularAssemblyToleranceUnits=rad  ConstraintSolverType=Machine precision  ConstraintRelTolerance=1e-4  ConstraintAbsTolerance=1e-4  UseRobustSingularityHandling=off  RedundancyAnalysisToleranceType=Automatically select tolerance  RedundancyAnalysisTolerance=1e-14  StatePerturbationType=Fixed  PerturbationSize=1e-5  VisualizeMachine=on
  Weld : mblibv1/Joints/Weld  DialogController=MECH.DynMechDlgSource  PhysicalDomain=mechanical  SubClassName=Unknown  LeftPortType=blob  RightPortType=blob  LConnTagsString=__newl0  RConnTagsString=__newr0  NumSAPorts=0  CutJoint=off  MarkAsCut=off  Primitives=weld  PrimitiveProps=W$INERTIAL$[0 0 0]$weld  DialogClass=JointBlock  WAxis=[0 0 0]
  TO CHASSIS : PMIOPort  Orientation=left  Port=1  Side=Right
  connections:
  Machine Environment/RConn1 -- Ground/LConn1
  Weld/LConn1 -- Ground/RConn1
  TO CHASSIS/RConn1 -- Weld/RConn1

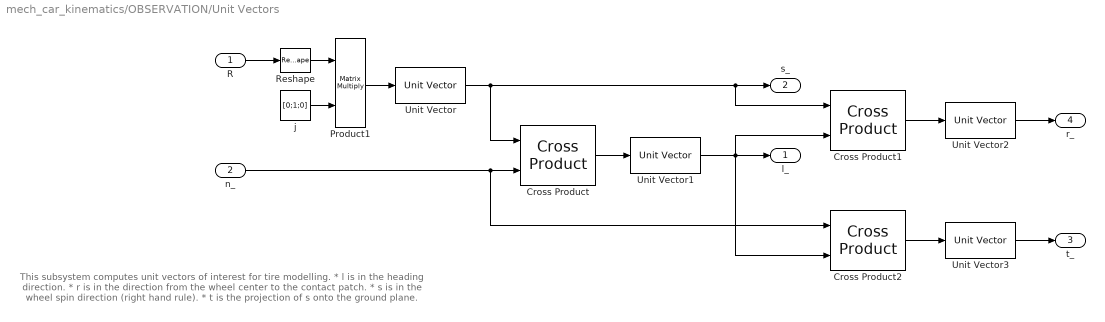
== system mech_car_kinematics/OBSERVATION/Unit Vectors ==
  note: This subsystem computes unit vectors of interest for tire modelling.
      | * l is in the heading direction.
      | * r is in the direction from the wheel center to the contact patch.
      | * s is in the wheel spin direction (right hand rule).
      | * t is the projection of s onto the ground plane.
  R : Inport  OutDataType=sfix(16)  OutScaling=2^0
  n_ : Inport  Port=2  OutDataType=sfix(16)  OutScaling=2^0
  Cross Product : mech_car_library/Utilities/Cross Product  SystemSampleTime=-1
  Cross Product1 : mech_car_library/Utilities/Cross Product  SystemSampleTime=-1
  Cross Product2 : mech_car_library/Utilities/Cross Product  SystemSampleTime=-1
  Product1 : Product  Multiplication=Matrix(*)  OutDataType=sfix(16)  OutScaling=2^0  RndMeth=Zero
  Reshape : Reshape  OutputDimensionality=Customize  OutputDimensions=[3,3]
  Unit Vector{,1..3} (4 alike) : mech_car_library/Utilities/Unit Vector  SystemSampleTime=-1
  j : Constant  Value=[0;1;0]  OutDataType=sfix(16)  OutScaling=2^0
  l_ : Outport  OutDataType=sfix(16)  OutScaling=2^0
  s_ : Outport  Port=2  OutDataType=sfix(16)  OutScaling=2^0
  t_ : Outport  Port=3  OutDataType=sfix(16)  OutScaling=2^0
  r_ : Outport  Port=4  OutDataType=sfix(16)  OutScaling=2^0
  wires:
  j/1 -> Product1/2
  R/1 -> Reshape/1
  Reshape/1 -> Product1/1
  Product1/1 -> Unit Vector/1
  Unit Vector/1 -> s_/1, Cross Product1/1, Cross Product/1
  Cross Product2/1 -> Unit Vector3/1
  Unit Vector3/1 -> t_/1
  Cross Product1/1 -> Unit Vector2/1
  Unit Vector2/1 -> r_/1
  n_/1 -> Cross Product/2, Cross Product2/1
  Cross Product/1 -> Unit Vector1/1
  Unit Vector1/1 -> l_/1, Cross Product1/2, Cross Product2/2

== system mech_car_kinematics/OBSERVATION/WHEEL LOCATION ==
